simulink model "PID_ADRC"  (R2022a)
settings: Solver=ode4  StartTime=0.0  StopTime=14.895  FixedStep=0.003  RelTol=1e-3
InitFcn:
  | T_set=2;
  | b0=1/(13.1);
  | T_sam=0.003;
  | s_cl=-6/T_set;
  | s_eso=1.5*s_cl;
  | z_eso=exp(s_eso*T_sam);
  | Kd=-2*s_cl;
  | Kp=(s_cl)^2;
  | l1=-3*s_eso;
  | l2=3*(s_eso)^2;
  | l3=-(s_eso)^3;
  | 
  | 
  | %Thong so Notch filter
  | w0=4.337;
  | D=0.0001;
  | T_set1=3;
  | b01=1/(0.87);
  | T_sam1=0.003;
  | s_cl1=-6/T_set1;
  | s_eso1=20*s_cl1;
  | z_eso1=exp(s_eso1*T_sam1);
  | Kd1=-2*s_cl1;
  | Kp1=(s_cl1)^2;
  | l11=-3*s_eso1;
  | l21=3*(s_eso1)^2;
  | l31=-(s_eso1)^3;
StopFcn:
  | B = [100, 100, 600 300];
  | figure('Position', B);
  | figure(1)
  | hold on;
  | plot(out.tout,out.F1,'linewidth',1.2);
  | %plot(out.tout,out.F11,'linewidth',1.2);
  | %plot(out.tout,out.F12,'linewidth',1.2);
  | %plot(out.tout,out.F13,'linewidth',1.2);
  | legend('PID');
  | xlabel('Thời gian (s)');
  | ylabel('F1 (N)');
  | grid on
  | 
  | % do thi vi tri
  | figure('Position', B);
  | figure(2)
  | plot(out.tout,out.X1,'linewidth',1.2);
  | %plot(out.tout,out.X11,'linewidth',1.2);
  | %plot(out.tout,out.X12,'linewidth',1.2);
  | %plot(out.tout,out.X13,'linewidth',1.2);
  | hold on
  | grid on
  | xlabel('Thời gian (s)');
  | ylabel('x1 (m)');
  | legend('PID);
  | 
  | % do thi dao dong diem giua
  | figure('Position', B);
  | figure(3)
  | hold on
  | grid on
  | plot(out.tout,out.W_MID,'linewidth',1.2);
  | %plot(out.tout,out.W_MID1,'--r','linewidth',1.2);
  | %plot(out.tout,out.W_MID2,'-.k','linewidth',1.2);
  | %plot(out.tout,out.W_MID3,'-m','linewidth',1.2);
  | xlabel('Thời gian (s)');
  | ylabel('ω(L/2, t)(m)');
  | legend('ADRC', 'ADRC+ZV','ADRC+ZVD','ADRC+ETM4');
  | 
  | % do thi dao dong diem cuoi
  | figure('Position', B);
  | figure(4)
  | hold on
  | grid on
  | plot(out.tout,out.WL,'linewidth',0.7);
  | %plot(out.tout,out.WL1,'linewidth',0.7);
  | %plot(out.tout,out.WL2,'linewidth',0.7);
  | %plot(out.tout,out.WL3,'linewidth',0.7);
  | xlabel('Thời gian (s)');
  | ylabel('ω(L,t) (m)');
  | legend('Middle point','End point');
  | axis([0 15 -0.04 0.04])
  | legend('ADRC', 'ADRC+ZV','ADRC+ZVD','ADRC+ETM4');
  | 
  | %do thi pho tan so
  | figure('Position', B);
  | tmax = 15;
  | r = 5000;
  | dt = tmax/(r);
  | Fs=1/dt;
  | time=0:dt:(r-2)*dt-dt;
  | l1=r;
  | grid on
  | hold on
  | 
  | fft_w=fft(out.W_MID,l1)*(2/l1);
  | abs_w=abs(fft_w);
  | freq=0:(1/time(end)):Fs/2-(1/time(end));
  | plot(freq,abs_w(1:length(freq)),LineWidth=1.2);
  | 
  | fft_w=fft(out.WL,l1)*(2/l1);
  | abs_w=abs(fft_w);
  | freq=0:(1/time(end)):Fs/2-(1/time(end));
  | plot(freq,abs_w(1:length(freq)),LineWidth=1.2);
  | xlabel('Tần số (Hz)');
  | ylabel('Biên độ (m)')
  | legend('Middle point','End point');
  | A = [0 10 0 0.02 ];
  | axis(A);
libraries: slpidlib x1
settings Model: Creator=Admin  LastModifiedBy=ducdu
settings DebuggingCC: UnconnectedInputMsg=warning  UnconnectedOutputMsg=warning  UnconnectedLineMsg=warning
settings RTWCC: DLArmComputeVersion=19.05

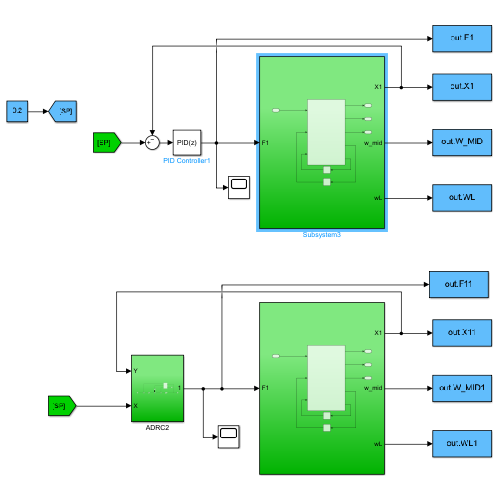
[thumbnail: Simulink's stored preview of the top-level diagram]
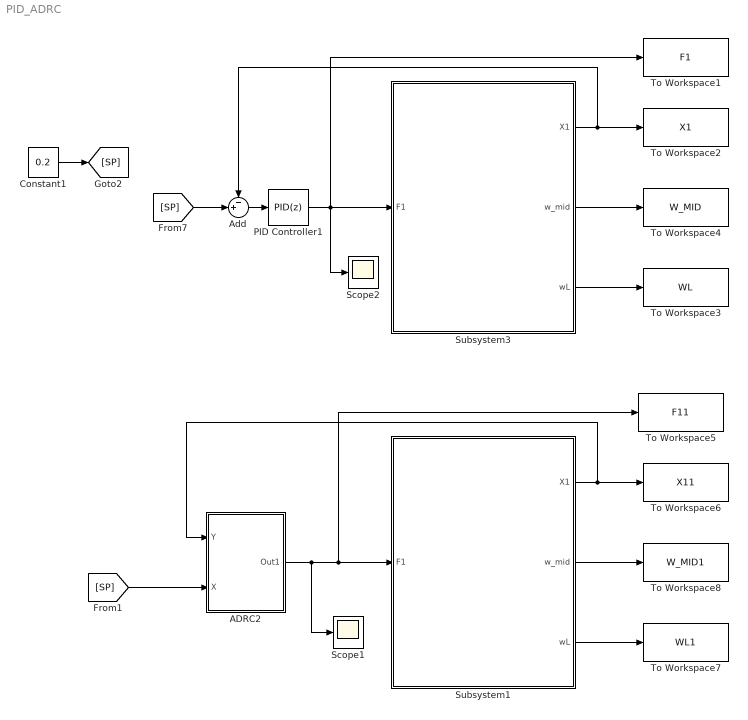
== system PID_ADRC ==
  ADRC2 : Subsystem
  Add : Sum  Inputs=-+|
  Constant1 : Constant  Value=0.2
  PID Controller1 : slpidlib/PID Controller  Controller=PID  Form=Parallel  TimeDomain=Discrete-time  UseExternalTs=off  SampleTime=0.003  IntegratorMethod=Forward Euler  FilterMethod=Forward Euler  ControllerParametersSource=internal  P=0.18380080341484  I=0.00264427661684036  UseKiTs=off  D=14.3583596221209  N=105.481990683281  UseFilter=on  TunerSelectOption=Transfer Function Based (PID Tuner App)  InitialConditionSource=internal  InitialConditionForIntegrator=0  InitialConditionForFilter=0  DifferentiatorICPrevScaledInput=0  ExternalReset=none  TrackingMode=off  Kt=1  LimitOutput=off  SatLimitsSource=internal  UpperSaturationLimit=inf  LowerSaturationLimit=-inf  LinearizeAsGain=on  AntiWindupMode=none  Kb=1  POutMin=[]  POutMax=[]  IOutMin=[]  IOutMax=[]  DOutMin=[]  DOutMax=[]  NOutMin=[]  NOutMax=[]  SumOutMin=[]  SumOutMax=[]  SaturationOutMin=[]  SaturationOutMax=[]  PParamMin=[]  PParamMax=[]  IParamMin=[]  IParamMax=[]  DParamMin=[]  DParamMax=[]  NParamMin=[]  NParamMax=[]  KbParamMin=[]  KbParamMax=[]  KtParamMin=[]  KtParamMax=[]  KbOutMin=[]  KbOutMax=[]  KtOutMin=[]  KtOutMax=[]  IntegratorOutMin=[]  IntegratorOutMax=[]  FilterOutMin=[]  FilterOutMax=[]  SumI1OutMin=[]  SumI1OutMax=[]  SumI2OutMin=[]  SumI2OutMax=[]  SumI3OutMin=[]  SumI3OutMax=[]  SumI4OutMin=[]  SumI4OutMax=[]  SumDOutMin=[]  SumDOutMax=[]  DifferentiatorOutMin=[]  DifferentiatorOutMax=[]  FilterDiffOutCoefMin=[]  FilterDiffOutCoefMax=[]  ReciprocalOutMin=[]  ReciprocalOutMax=[]  SumDenOutMin=[]  SumDenOutMax=[]  SumNumOutMin=[]  SumNumOutMax=[]  DivideOutMin=[]  DivideOutMax=[]  UdiffTsProdOutMin=[]  UdiffTsProdOutMax=[]  NTsProdOutMin=[]  NTsProdOutMax=[]  UintegralTsProdOutMin=[]  UintegralTsProdOutMax=[]  UngainTsProdOutMin=[]  UngainTsProdOutMax=[]  IntegratorContinuousStateAttributes=''  IntegratorStateMustResolveToSignalObject=off  IntegratorRTWStateStorageClass=Auto  FilterContinuousStateAttributes=''  FilterStateMustResolveToSignalObject=off  FilterRTWStateStorageClass=Auto  ParallelPVariant=InternalParameters  IdealPVariant=Disabled  IVariant=InternalParameters  DVariant=InternalParameters  IntegratorVariant=Discrete  SatVariant=Disabled  AWVariant=Passthrough  PCopyVariant=Disabled  TRVariant=Disabled  FdbkBlocksVariant=Forward  IdealPFdbkVariant=Disabled  SatFdbkVariant=Disabled  DerivativeFilterVariant=ForwardEulerFilter  NVariant=InternalParameters  NCopyVariant=Disabled  FilterICVariant=InternalICsFilter  IntegratorICVariant=InternalICs  ExternalResetVariant=Disabled  TRSumVariant=Passthrough  SumFdbkVariant=Disabled  SumVariant=Sum_PID  TsampFilterVariant=InternalTs  TsampNgainVariant=Passthrough  TsampIntegralVariant=Passthrough  ExternalSaturationOutDataTypeStr=Inherit: Same as second input  aMode=0
  Scope1 : Scope
  Scope2 : Scope
  Subsystem1 : Subsystem
  Subsystem3 : Subsystem
  To Workspace1 : ToWorkspace  VariableName=F1  SampleTime=-1
      settings: Save2DSignal=2-D array (concatenate along first dimension)
  To Workspace2 : ToWorkspace  VariableName=X1  SampleTime=-1
      settings: Save2DSignal=2-D array (concatenate along first dimension)
  To Workspace3 : ToWorkspace  VariableName=WL  SampleTime=-1
      settings: Save2DSignal=2-D array (concatenate along first dimension)
  To Workspace4 : ToWorkspace  VariableName=W_MID  SampleTime=-1
      settings: Save2DSignal=2-D array (concatenate along first dimension)
  To Workspace5 : ToWorkspace  VariableName=F11  SampleTime=-1
      settings: Save2DSignal=2-D array (concatenate along first dimension)
  To Workspace6 : ToWorkspace  VariableName=X11  SampleTime=-1
      settings: Save2DSignal=2-D array (concatenate along first dimension)
  To Workspace7 : ToWorkspace  VariableName=WL1  SampleTime=-1
      settings: Save2DSignal=2-D array (concatenate along first dimension)
  To Workspace8 : ToWorkspace  VariableName=W_MID1  SampleTime=-1
      settings: Save2DSignal=2-D array (concatenate along first dimension)
  wires:
  Subsystem3/1(X1) -> Add/1, To Workspace2/1
  [SP] -> Add/2
  Constant1/1 -> [SP]
  Subsystem3/2(w_mid) -> To Workspace4/1
  Subsystem3/3(wL) -> To Workspace3/1
  Add/1 -> PID Controller1/1
  PID Controller1/1 -> To Workspace1/1, Subsystem3/1(F1), Scope2/1
  Subsystem1/3(wL) -> To Workspace7/1
  Subsystem1/1(X1) -> ADRC2/1(Y), To Workspace6/1
  Subsystem1/2(w_mid) -> To Workspace8/1
  ADRC2/1(Out1) -> To Workspace5/1, Subsystem1/1(F1), Scope1/1
  [SP] -> ADRC2/2(X)

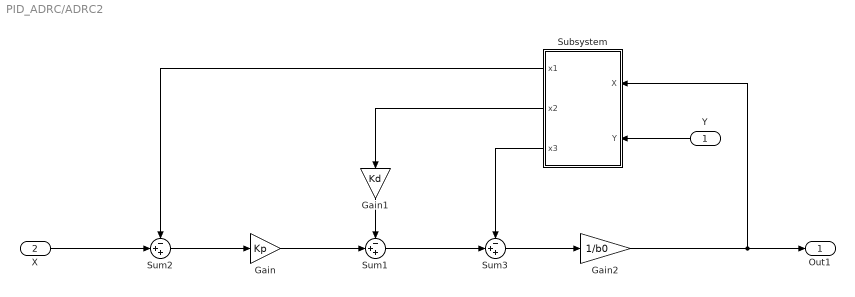
== system PID_ADRC/ADRC2 ==
  Y : Inport
  X : Inport  Port=2
  Gain : Gain  Gain=Kp
  Gain1 : Gain  Gain=Kd
  Gain2 : Gain  Gain=1/b0
  Subsystem : Subsystem
  Sum1 : Sum  Inputs=-++
  Sum2 : Sum  Inputs=-++
  Sum3 : Sum  Inputs=-++
  Out1 : Outport
  wires:
  Sum1/1 -> Sum3/2
  Subsystem/1(x1) -> Sum2/1
  Sum3/1 -> Gain2/1
  Gain/1 -> Sum1/2
  Subsystem/3(x3) -> Sum3/1
  Gain1/1 -> Sum1/1
  Gain2/1 -> Out1/1, Subsystem/1(X)
  Subsystem/2(x2) -> Gain1/1
  Sum2/1 -> Gain/1
  Y/1 -> Subsystem/2(Y)
  X/1 -> Sum2/2

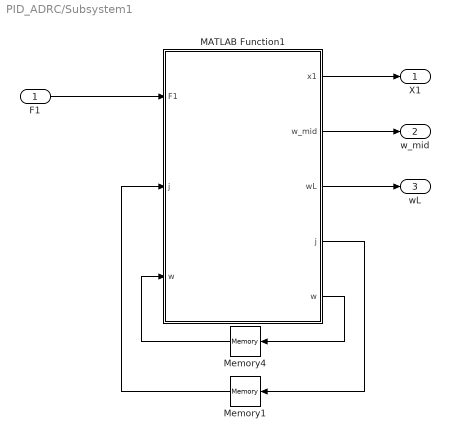
== system PID_ADRC/Subsystem1 ==
  F1 : Inport
  MATLAB Function1 : MATLAB Function  TreatAsAtomicUnit=on
  Memory1 : Memory
  Memory4 : Memory  InitialCondition=zeros(15,10000)
  X1 : Outport
  w_mid : Outport  Port=2
  wL : Outport  Port=3
  wires:
  Memory4/1 -> MATLAB Function1/3("w ")
  Memory1/1 -> MATLAB Function1/2("j ")
  MATLAB Function1/4(j) -> Memory1/1
  MATLAB Function1/5(w) -> Memory4/1
  MATLAB Function1/3(wL) -> wL/1
  F1/1 -> MATLAB Function1/1(F1)
  MATLAB Function1/1(x1) -> X1/1
  MATLAB Function1/2(w_mid) -> w_mid/1

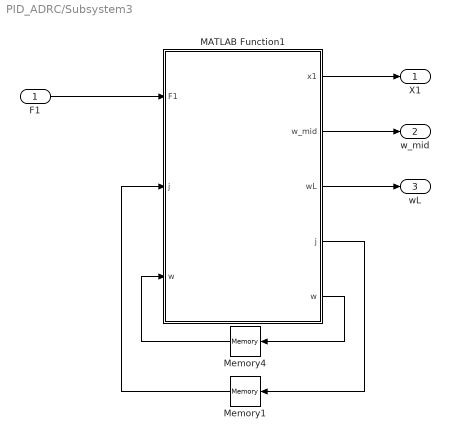
== system PID_ADRC/Subsystem3 ==
  F1 : Inport
  MATLAB Function1 : MATLAB Function  TreatAsAtomicUnit=on
  Memory1 : Memory
  Memory4 : Memory  InitialCondition=zeros(15,10000)
  X1 : Outport
  w_mid : Outport  Port=2
  wL : Outport  Port=3
  wires:
  Memory4/1 -> MATLAB Function1/3("w ")
  Memory1/1 -> MATLAB Function1/2("j ")
  MATLAB Function1/4(j) -> Memory1/1
  MATLAB Function1/5(w) -> Memory4/1
  MATLAB Function1/3(wL) -> wL/1
  F1/1 -> MATLAB Function1/1(F1)
  MATLAB Function1/1(x1) -> X1/1
  MATLAB Function1/2(w_mid) -> w_mid/1

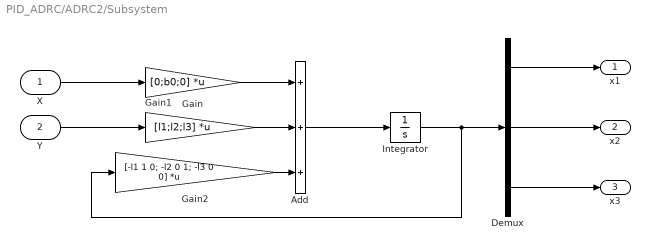
== system PID_ADRC/ADRC2/Subsystem ==
  X : Inport
  Y : Inport  Port=2
  Add : Sum  Inputs=+++
  Demux : Demux  Outputs=3
  Gain : Gain  Gain=[0;b0;0]  Multiplication=Matrix(K*u)
  Gain1 : Gain  Gain=[l1;l2;l3]  Multiplication=Matrix(K*u)
  Gain2 : Gain  Gain=[-l1 1 0; -l2 0 1; -l3 0 0]  Multiplication=Matrix(K*u)
  Integrator : Integrator
  x1 : Outport
  x2 : Outport  Port=2
  x3 : Outport  Port=3
  wires:
  Gain1/1 -> Add/2
  Demux/3 -> x3/1
  Demux/1 -> x1/1
  Gain2/1 -> Add/3
  Demux/2 -> x2/1
  Gain/1 -> Add/1
  Add/1 -> Integrator/1
  Integrator/1 -> Gain2/1, Demux/1
  Y/1 -> Gain1/1
  X/1 -> Gain/1

== matlab function PID_ADRC/Subsystem1/MATLAB Function1 ==
  data: F1 input; x1 output; w_mid output; wL output; j input; j output; w input; w output
function [x1,w_mid,wL,j,w]= fcn(F1,j,w)
%nhap so lieu cua dam`
k=1;
pA=2.4882;EI=0.236;g=9.81;
%pA=2.4882;EI=0.1635;g=9.81;
% pA=2.4882;EI=1.05;g=9.81;
L=0.6;
mw=13.1;
mk=0.2;
% cac buoc sai phan
tmax=15;
r=5000;
dt=tmax/r;
n=9;% so diem chia => chia thanh thanh 5 diem 
ds=L/(n-1); 
S1=(EI*(dt^2))/(mw*(ds^3));
S2=(-EI*(dt^2))/((ds^4)*pA);
S3=(EI*(dt^2))/(mk*2*ds^3);
j=j+1;
% mo phong diem x1
S1=(EI*dt^2)/(mw*ds^3);
wsss01=(w(3,j+1)-2*w(2,j+1)+w(1,j+1))/(2*ds^3);
w(1,j+2)=(F1-EI*wsss01)*(dt^2/mw)+2*w(1,j+1)-w(1,j);
w(2,j+2)=w(1,j+2);
for i=3:n-2
S2=(-EI*dt^2)/(ds^4*pA);
wssss=w(i+2,j+1)-4*w(i+1,j+1)+6*w(i,j+1)-4*w(i-1,j+1)+w(i-2,j+1);
w(i,j+2)=S2*wssss+2*w(i,j+1)-w(i,j);
end
wsssl=(-2*w(n,j+1)+3*w(n-1,j+1)-w(n-2,j+1));
w(n,j+2)=2*w(n,j+1)-w(n,j)+S3*wsssl;
w(n-1,j+2)=(w(n,j+2)+w(n-2,j+2))/2;
x1=w(1,j);
wL=w(n,j)-w(1,j);
w_mid=w(5,j)-w(1,j);
end

== matlab function PID_ADRC/Subsystem3/MATLAB Function1 ==
  data: F1 input; x1 output; w_mid output; wL output; j input; j output; w input; w output
function [x1,w_mid,wL,j,w]= fcn(F1,j,w)
%nhap so lieu cua dam`
pA=2.4882;EI=0.236;
%pA=2.4882;EI=0.1635;g=9.81;
% pA=2.4882;EI=1.05;g=9.81;
L=0.6;
mw=13.1;
mk=0.2;
% cac buoc sai phan
tmax=15;
r=5000;
dt=tmax/r;
n=9;% so diem chia => chia thanh thanh 5 diem 
ds=L/(n-1); 
S3=(EI*(dt^2))/(mk*2*ds^3);
j = j + 1;
% mo phong diem x1
wsss01=(w(3,j+1)-2*w(2,j+1)+w(1,j+1))/(2*ds^3);
w(1,j+2)=(F1-EI*wsss01)*(dt^2/mw)+2*w(1,j+1)-w(1,j);
w(2,j+2)=w(1,j+2);
for i=3:n-2
S2=(-EI*dt^2)/(ds^4*pA);
wssss=w(i+2,j+1)-4*w(i+1,j+1)+6*w(i,j+1)-4*w(i-1,j+1)+w(i-2,j+1);
w(i,j+2)=S2*wssss+2*w(i,j+1)-w(i,j);
end
wsssl=(-2*w(n,j+1)+3*w(n-1,j+1)-w(n-2,j+1));
w(n,j+2)=2*w(n,j+1)-w(n,j)+S3*wsssl;
w(n-1,j+2)=(w(n,j+2)+w(n-2,j+2))/2;
x1=w(1,j);
wL=w(n,j)-w(1,j);
w_mid=w(5,j)-w(1,j);
end
